simulink model "AugmentedConstrainted"  (R2013a)
settings: Solver=ode45  StartTime=0.0  StopTime=10.0  RelTol=1e-3
settings Model: Creator=G.force  LastModifiedBy=G.force

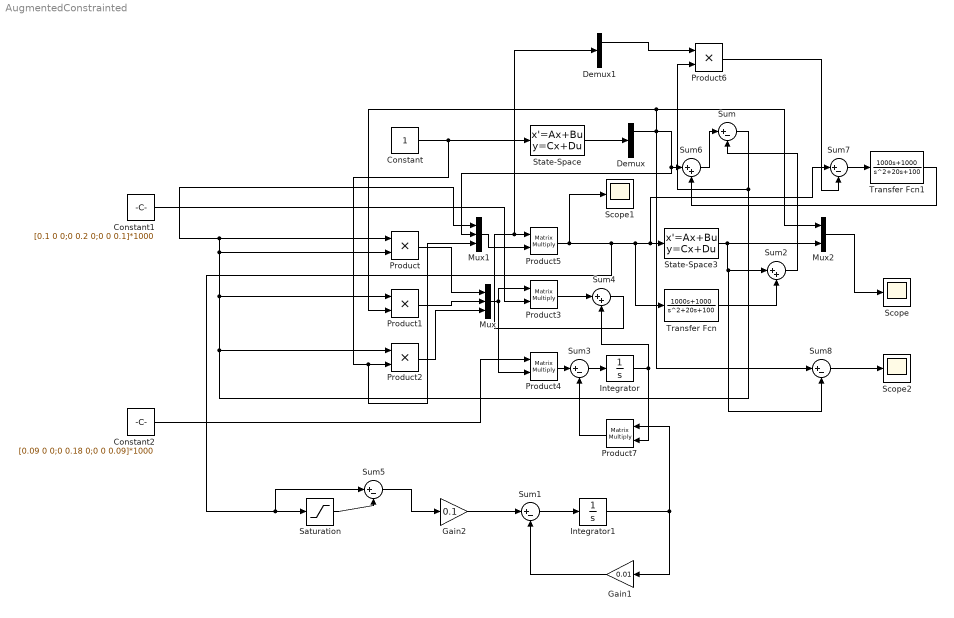
== system AugmentedConstrainted ==
  Constant : Constant
  Constant1 : Constant  Value=[0.1 0 0;0 0.2 0;0 0 0.1]*1000
  Constant2 : Constant  Value=[0.09 0 0;0 0.18 0;0 0 0.09]*1000
  Demux : Demux  Outputs=2
  Demux1 : Demux  Outputs=3
  Gain1 : Gain  Gain=0.01
  Gain2 : Gain  Gain=0.1
  Integrator : Integrator  InitialCondition=[0.01 0.020841 1e-6]
  Integrator1 : Integrator
  Mux : Mux  Inputs=3
  Mux1 : Mux  Inputs=3
  Mux2 : Mux  Inputs=2
  Product{,1..2,6} (4 alike) : Product
  Product{3..5,7} (4 alike) : Product  Multiplication=Matrix(*)
  Saturation : Saturate  UpperLimit=0.001  LowerLimit=-0.001
  Scope : Scope
      settings: ShowLegends=on  TimeRange=4  YMin=-40  YMax=45  SaveName=sd  MaxDataPoints=100000000
  Scope1 : Scope
      settings: TimeRange=10  SaveName=Up  MaxDataPoints=100000000
  Scope2 : Scope
      settings: ShowLegends=on  TimeRange=4  YMin=-40  YMax=45  SaveName=E  MaxDataPoints=10000000
  State-Space : StateSpace  A=[-1 0;0 -1]  B=[1;1]  C=eye(2)  D=[0;0]  X0=[0 0]
  State-Space3 : StateSpace  A=[0 1;-2084.1 0]  B=[0;0.9999]*1e5  C=[1 0]  D=0
  Sum{,1,3,5,7..8} (6 alike) : Sum  Inputs=|+-
  Sum2 : Sum  Inputs=|++
  Sum4 : Sum  Inputs=|++
  Sum6 : Sum  Inputs=|++
  Transfer Fcn : TransferFcn  Numerator=[1000 1000]  Denominator=[1 20 100]
  Transfer Fcn1 : TransferFcn  Numerator=[1000 1000]  Denominator=[1 20 100]
  wires:
  Constant/1 -> Mux1/3, Product2/2, State-Space/1
  Sum/1 -> Product6/2, Product2/1, Product1/1, Product/2, Product/1, Mux1/1
  Product/1 -> Mux/1
  Product1/1 -> Mux/2
  Product2/1 -> Mux/3
  Mux/1 -> Product3/1, Product4/2
  Constant1/1 -> Product3/2
  Constant2/1 -> Product4/1
  Product4/1 -> Sum3/1
  Sum3/1 -> Integrator/1
  Product3/1 -> Sum4/1
  Sum4/1 -> Demux1/1, Product5/1
  Mux1/1 -> Product5/2
  Mux2/1 -> Scope/1
  Integrator1/1 -> Gain1/1, Product7/1
  Integrator/1 -> Sum4/2, Product7/2
  State-Space3/1 -> Sum8/2, Sum2/1, Mux2/2
  Gain1/1 -> Sum1/2
  Sum1/1 -> Integrator1/1
  Saturation/1 -> Sum5/2
  Product5/1 -> Scope1/1, Sum5/1, Saturation/1, Transfer Fcn/1, Sum7/1, State-Space3/1
  Sum5/1 -> Gain2/1
  State-Space/1 -> Demux/1
  Gain2/1 -> Sum1/1
  Transfer Fcn/1 -> Sum2/2
  Sum2/1 -> Sum/2
  Demux/1 -> Sum8/1, Product1/2, Mux2/1, Mux1/2, Sum6/1
  Transfer Fcn1/1 -> Sum6/2
  Sum6/1 -> Sum/1
  Demux1/1 -> Product6/1
  Sum7/1 -> Transfer Fcn1/1
  Product6/1 -> Sum7/2
  Sum8/1 -> Scope2/1
  Product7/1 -> Sum3/2
